simulink model "method2"  (R2023b)
settings: Solver=ode4  StartTime=0.0  StopTime=10.0  FixedStep=0.001  RelTol=1e-3
InitFcn:
  | constants_pend
values from neighbouring files (symbols this model uses):
  f = 2    [constants_pend.m]    (also in formethod3.m = u(1))
  initial = [0.5 , 5 , pi/3 , 0 ]    [constants_pend.m]
settings Model: Creator=User  LastModifiedBy=User

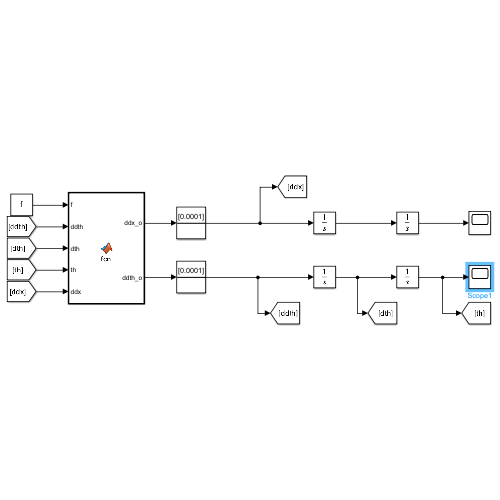
[thumbnail: Simulink's stored preview of the top-level diagram]
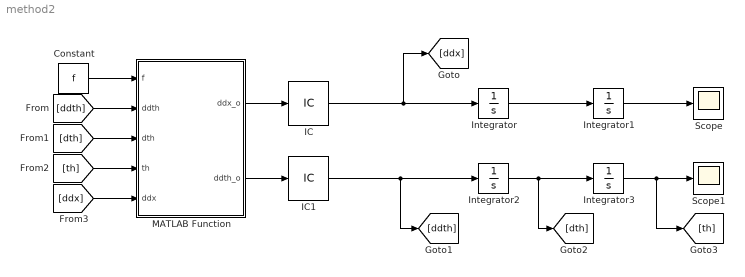
== system method2 ==
  Constant : Constant  Value=f
  IC : InitialCondition  Value=0.0001
  IC1 : InitialCondition  Value=0.0001
  Integrator : Integrator  InitialCondition=initial(2)
  Integrator1 : Integrator  InitialCondition=initial(1)
  Integrator2 : Integrator  InitialCondition=initial(4)
  Integrator3 : Integrator  InitialCondition=initial(3)
  MATLAB Function : MATLAB Function  TreatAsAtomicUnit=on
  Scope : Scope
  Scope1 : Scope
  wires:
  MATLAB Function/1(ddx_o) -> IC/1
  Integrator/1 -> Integrator1/1
  Integrator1/1 -> Scope/1
  Integrator3/1 -> [th], Scope1/1
  Integrator2/1 -> [dth], Integrator3/1
  MATLAB Function/2(ddth_o) -> IC1/1
  Constant/1 -> MATLAB Function/1(f)
  [ddth] -> MATLAB Function/2(ddth)
  [dth] -> MATLAB Function/3(dth)
  [th] -> MATLAB Function/4(th)
  [ddx] -> MATLAB Function/5(ddx)
  IC/1 -> [ddx], Integrator/1
  IC1/1 -> [ddth], Integrator2/1

== matlab function method2/MATLAB Function ==
  data: f input; ddx_o output; ddth input; dth input; th input; ddx input; ddth_o output
function [ddx_o,ddth_o] = fcn(f,ddth,dth,th,ddx)
mp = 0.35;
mc = 2 ;
l = 0.75;
g = 9.81 ;

ddx_o = (f - mp*l*ddth*cos(th)  + mp*l*dth^2*sin(th) )  / (mc+mp) ;
ddth_o = ( - mp*l*ddx*cos(th) -  mp*l*g*sin(th)) / (mp*l^2);
